simulink model "MaxpidE_Modele_Causal_BO_Courant"  (R2024b)
settings: Solver=VariableStepAuto  StartTime=0.0  StopTime=1  RelTol=1e-3
InitFcn:
  | run('parametres.m')
values from neighbouring files (symbols this model uses):
  Cfs = 0.0328    [parametres.m]
  f = 0.0006    [parametres.m]
  Jm = 79e-3*1e-4    (= 7.9e-06)    [parametres.m]
  Jv = 10.8*Lv*1e-6    (= 3.24e-06)    [parametres.m]
  Kc = 29.2e-3    (= 0.0292)    [parametres.m]
  Ke = 1/Ke    (= 0.0291137091022)    [parametres.m]
  KI_i = 200    [parametres.m]
  KP_i = 800    [parametres.m]
  Lm = 0.191e-3    (= 0.000191)    [parametres.m]
  Rm = 0.582    [parametres.m]
  t_acc = theta_p / theta_pp    (= 0.277777777778)    [parametres.m]
  theta_p = 2.5    [parametres.m]
  Umax = 24    [parametres.m]
libraries: simulink x4
settings Model: Creator=xpess  LastModifiedBy=xpess
settings RTWCC: GPUComputeCapability=3.5

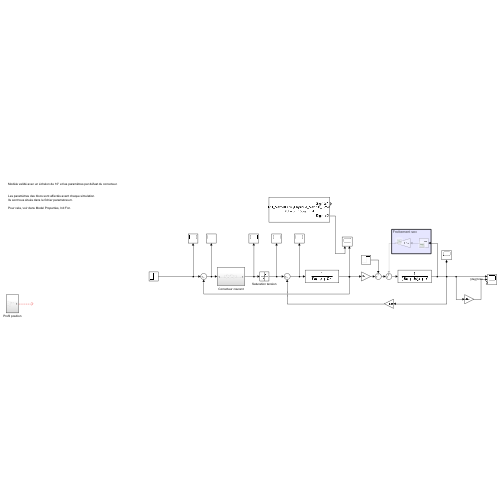
[thumbnail: Simulink's stored preview of the top-level diagram]
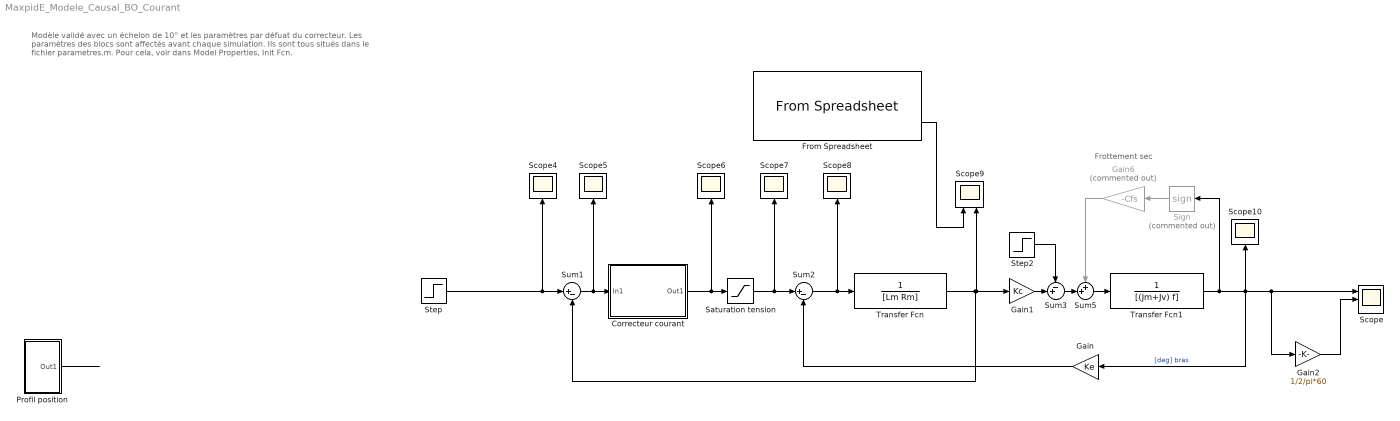
== system MaxpidE_Modele_Causal_BO_Courant ==
  note: Modèle validé avec un échelon de 10° et les paramètres par défuat du correcteur.
      |
      |
      | Les paramètres des blocs sont affectés avant chaque simulation.
      | Ils sont tous situés dans le fichier parametres.m.
      |
      | Pour cela, voir dans Model Properties, Init Fcn.
  note: Frottement sec
  Correcteur courant : Subsystem
  From Spreadsheet : FromSpreadsheet  FileName=C:\GitHub\TP_Documents_PSI\11_MaxpidE\PolyPhysique_MaxPID_E\Mesures\Echelon_10deg_I_H.xlsx  SheetName=Echelon_10deg_I_H  Range=A2:C103
  Gain : Gain  Gain=Ke
  Gain1 : Gain  Gain=Kc
  Gain2 : Gain  Gain=1/2/pi*60
  Gain6 : Gain  Commented=on  Gain=-Cfs
  Profil position : Subsystem
  Saturation tension : Saturate  UpperLimit=Umax  LowerLimit=-Umax
  Scope : Scope  NumInputPorts=3
  Scope{4..8,10} (6 alike) : Scope
  Scope9 : Scope  NumInputPorts=2
  Sign : Signum  Commented=on  ZeroCross=off
  Step : Step  Time=0  After=2.5  SampleTime=0
  Step2 : Step  After=0  SampleTime=0
  Sum1 : Sum  Inputs=|+-
  Sum2 : Sum  Inputs=|+-
  Sum3 : Sum  Inputs=-+|
  Sum5 : Sum  Inputs=++|
  Transfer Fcn : TransferFcn  Denominator=[Lm Rm]
  Transfer Fcn1 : TransferFcn  Denominator=[(Jm+Jv) f]
  wires:
  Correcteur courant/1(Out1) -> Scope6/1, Saturation tension/1
  Sum1/1 -> Scope5/1, Correcteur courant/1(In1)
  Step/1 -> Scope4/1, Sum1/1
  Saturation tension/1 -> Sum2/1, Scope7/1
  Sum2/1 -> Scope8/1, Transfer Fcn/1
  Transfer Fcn/1 -> Scope9/2, Gain1/1, Sum1/2
  Gain/1 -> Sum2/2
  Gain1/1 -> Sum3/2
  Transfer Fcn1/1 -> Sign/1, Scope10/1, Gain2/1, Scope/1, Gain/1  "[deg] bras"
  Step2/1 -> Sum3/1
  Profil position/1(Out1) -> ?
  Sum3/1 -> Sum5/2
  Sum5/1 -> Transfer Fcn1/1
  Sign/1 -> Gain6/1
  Gain6/1 -> Sum5/1
  From Spreadsheet/2 -> Scope9/1
  Gain2/1 -> Scope/2

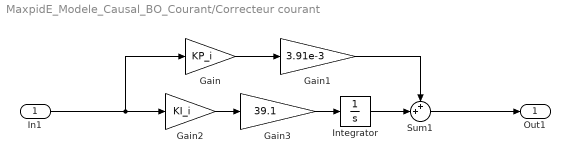
== system MaxpidE_Modele_Causal_BO_Courant/Correcteur courant ==
  In1 : Inport
  Gain : Gain  Gain=KP_i
  Gain1 : Gain  Gain=3.91e-3
  Gain2 : Gain  Gain=KI_i
  Gain3 : Gain  Gain=39.1
  Integrator : Integrator
  Sum1 : Sum  Inputs=++|
  Out1 : Outport
  wires:
  Sum1/1 -> Out1/1
  Gain3/1 -> Integrator/1
  Integrator/1 -> Sum1/2
  Gain2/1 -> Gain3/1
  In1/1 -> Gain2/1, Gain/1
  Gain/1 -> Gain1/1
  Gain1/1 -> Sum1/1

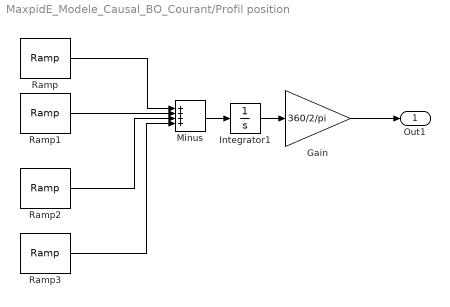
== system MaxpidE_Modele_Causal_BO_Courant/Profil position ==
  Gain : Gain  Gain=360/2/pi
  Integrator1 : Integrator
  Minus : Sum  Inputs=++++
  Ramp : simulink/Sources/Ramp  slope=theta_p/t_acc  start=t0  InitialOutput=0
  Ramp1 : simulink/Sources/Ramp  slope=-theta_p/t_acc  start=t1  InitialOutput=0
  Ramp2 : simulink/Sources/Ramp  slope=-theta_p/t_acc  start=t2  InitialOutput=0
  Ramp3 : simulink/Sources/Ramp  slope=theta_p/t_acc  start=t3  InitialOutput=0
  Out1 : Outport
  wires:
  Ramp/1 -> Minus/1
  Integrator1/1 -> Gain/1
  Ramp3/1 -> Minus/4
  Ramp1/1 -> Minus/2
  Ramp2/1 -> Minus/3
  Minus/1 -> Integrator1/1
  Gain/1 -> Out1/1
